simulink model "mfcm_siso_sim"  (Simulink 6.1)
settings: Solver=VariableStepDiscrete  StartTime=0.0  StopTime=150000  RelTol=1e-3
values from neighbouring files (symbols this model uses):
  j = find(xLabel==')')    [sdspfscope2_r13.m]
undefined symbols (not defined in the file or in its folder): calc_path_data
libraries: xbsIndex_r4 x23, simulink x5, xbsCopyrightNotice_r4 x1, xrbsComm_r4 x1, dspsigops x1, dspmathops x1
settings Model: Creator=singhj  LastModifiedBy=alexc
settings DebuggingCC: SolverPrmCheckMsg=warning

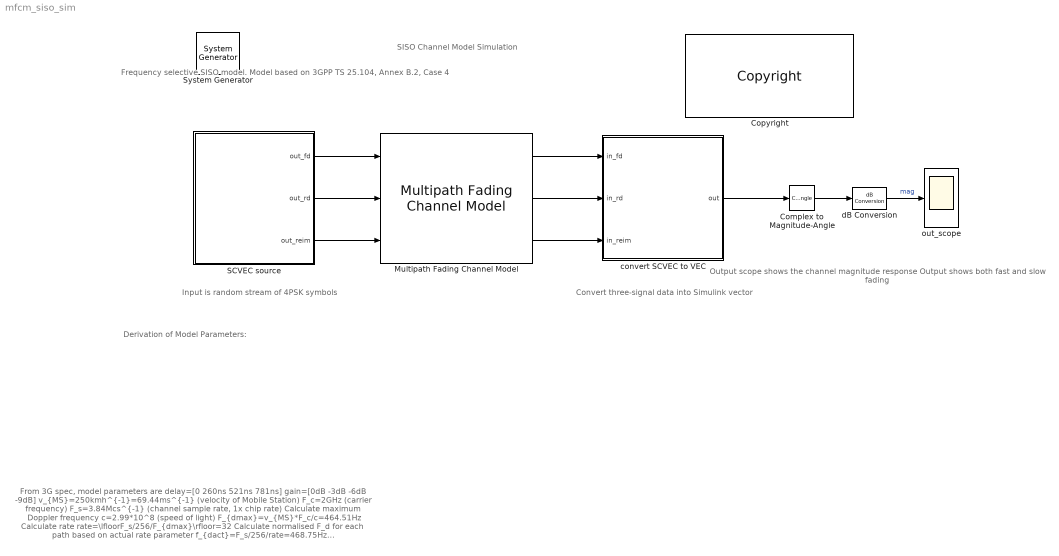
== system mfcm_siso_sim ==
  note: Output scope shows the channel magnitude response
      |
      | Output shows both fast and slow fading
  note: From 3G spec, model parameters are
      |   delay=[0 260ns 521ns 781ns]
      |   gain=[0dB -3dB -6dB -9dB]
      |   v_{MS}=250kmh^{-1}=69.44ms^{-1} (velocity of Mobile Station)
      |   F_c=2GHz (carrier frequency)
      |   F_s=3.84Mcs^{-1} (channel sample rate, 1x chip rate)
      |
      | Calculate maximum Doppler frequency
      |   c=2.99*10^8 (speed of light)
      |   F_{dmax}=v_{MS}*F_c/c=464.51Hz
      |
      | Calculate rate
      |   rate=\lfloorF_s/256/F_{dmax}\rfloor=32
      |
      | Calculate normalised F_d for each path based on actual rate parameter
      |   f_{dact}=F_s/256/rate=468.75Hz
      |   f_d=F_{dmax}/F_{dact}=0.990
      |
      | This can be passed as the second parameter of 'calc\_path\_data' to correct for the small difference between specified and actual F_d
      |   calc\_path\_data(ones(1,1,4)*2,0.990)
      |
      | Convert the delay vector to sample indexes
      |   delay_{sam}=round(delay*F_s)=[0 1 2 3]
      |
      | Convert the gain vector from dB to linear
      |   gain_{linear}=10^{gain/10}=[1.000 0.5012 0.2512 0.1259]
  note: SISO Channel Model Simulation
  note: Input is random stream of 4PSK symbols
  note: Convert three-signal data into
      | Simulink vector
  note: Frequency selective SISO model. Model based on 3GPP TS 25.104, Annex B.2, Case 4
  note: Derivation of Model Parameters:
  " System Generator" : xbsIndex_r4/ System Generator  Tag=genX  xilinxfamily=Virtex4  part=xc4vsx25  speed=-11  package=ff668  synthesis_tool=XST  directory=./netlist  testbench=off  simulink_period=1  sysclk_period=5  incr_netlist=off  trim_vbits=Everywhere in SubSystem  dbl_ovrd=According to Block Masks  core_generation=According to Block Masks  run_coregen=off  deprecated_control=off  eval_field=0  block_type=sysgen
  Complex to Magnitude-Angle : ComplexToMagnitudeAngle  Output=Magnitude
  Copyright : xbsCopyrightNotice_r4/Copyright
  Multipath Fading Channel Model : xrbsComm_r4/Multipath Fading Channel Model  DELAY=[0; 1; 2; 3]  GAIN=10.^([0; -3; -6; -9]/10)  RT=1  RR=1  SPEC_DATA=calc_path_data(ones(1,1,4)*2,0.990)  RATE=32  DATAPATH_WIDTH=18  TX_BINPT=17  FADE_BINPT=15  RX_BINPT=15  MAT_BINPT=17  SEED='461AF8228C9F8C92'  block_type=delay
      settings: infoedit=Multipath Fading Channel Model.  block_version=VER_STRING_GOES_HERE
  SCVEC source : Subsystem  mask{DATA=exp(j*2*pi*(round(4*rand(1,8191))+0.5)/4), WIDTH=18, BINPT=17, TF=2*4*1*1*ceil(64/32), REP_FILL=Zeros, TS=1}
      mask prompts: DATA "Constant Data"; WIDTH "Output Width"; BINPT "Output Binary Point"; TF "Frame Period (fd-to-fd time)"; REP_FILL "Fill with:"; TS "Sample Period"
      mask StyleString: edit,edit,edit,edit,popup(Zeros|Data),edit
  convert SCVEC to VEC : Subsystem  mask{VEC_SIZE=1, REP=1}
      mask prompts: VEC_SIZE "Input Vector Size"; REP "Output Repetition Count"
  dB Conversion : dspmathops/dB Conversion  dBtype=dB  intype=Amplitude  R=1  fuzz=off
  out_scope : Scope
      settings: YMin=-40  YMax=20  MaxDataPoints=150000
  wires:
  Complex to Magnitude-Angle/1 -> dB Conversion/1
  dB Conversion/1 -> out_scope/1  "mag"
  SCVEC source/1(out_fd) -> Multipath Fading Channel Model/1
  SCVEC source/2(out_rd) -> Multipath Fading Channel Model/2
  SCVEC source/3(out_reim) -> Multipath Fading Channel Model/3
  convert SCVEC to VEC/1(out) -> Complex to Magnitude-Angle/1
  Multipath Fading Channel Model/1 -> convert SCVEC to VEC/1(in_fd)
  Multipath Fading Channel Model/2 -> convert SCVEC to VEC/2(in_rd)
  Multipath Fading Channel Model/3 -> convert SCVEC to VEC/3(in_reim)

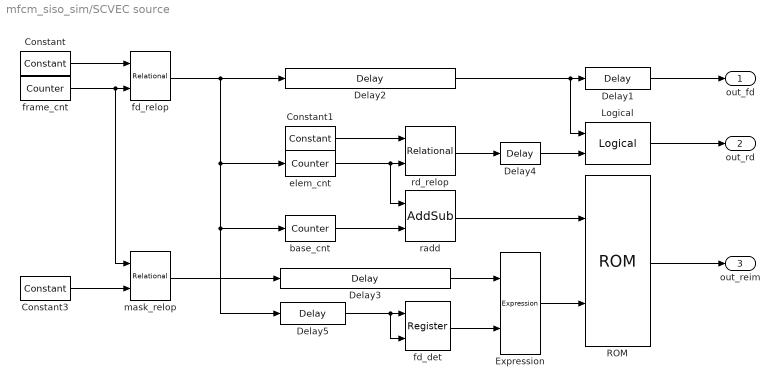
== system mfcm_siso_sim/SCVEC source ==
  Constant : xbsIndex_r4/Constant  arith_type=Unsigned  const=0  n_bits=1  bin_pt=0  explicit_period=off  period=1  equ=P=C  opselect=C  inp2=PCIN>>17  opr=+  inp1=P  carry=CIN  dbl_ovrd=off  block_type=constant
      settings: block_version=VER_STRING_GOES_HERE
  Constant1 : xbsIndex_r4/Constant  arith_type=Unsigned  const=2*size(DATA,1)-1  n_bits=ceil(log2(2*size(DATA,1)))  bin_pt=0  explicit_period=off  period=1  equ=P=C  opselect=C  inp2=PCIN>>17  opr=+  inp1=P  carry=CIN  dbl_ovrd=off  block_type=constant
      settings: block_version=VER_STRING_GOES_HERE
  Constant3 : xbsIndex_r4/Constant  arith_type=Unsigned  const=2*size(DATA,1)*double(REP_FILL==1)+TF*double(REP_FILL==2)  n_bits=1+ceil(log2(TF))  bin_pt=0  explicit_period=off  period=1  equ=P=C  opselect=C  inp2=PCIN>>17  opr=+  inp1=P  carry=CIN  dbl_ovrd=off  block_type=constant
      settings: block_version=VER_STRING_GOES_HERE
  Delay1 : xbsIndex_r4/Delay  en=off  latency=1  dbl_ovrd=off  reg_retiming=off  block_type=delay
      settings: infoedit=Hardware notes: A delay line is a chain, each link of which is an SRL16 followed by a flip-flop. If register retiming is enabled, the delay line is a chain of flip-flops.  block_version=VER_STRING_GOES_HERE
  Delay2 : xbsIndex_r4/Delay  en=off  latency=2  dbl_ovrd=off  reg_retiming=off  block_type=delay
      settings: infoedit=Hardware notes: A delay line is a chain, each link of which is an SRL16 followed by a flip-flop. If register retiming is enabled, the delay line is a chain of flip-flops.  block_version=VER_STRING_GOES_HERE
  Delay3 : xbsIndex_r4/Delay  en=off  latency=2  dbl_ovrd=off  reg_retiming=off  block_type=delay
      settings: infoedit=Hardware notes: A delay line is a chain, each link of which is an SRL16 followed by a flip-flop. If register retiming is enabled, the delay line is a chain of flip-flops.  block_version=VER_STRING_GOES_HERE
  Delay4 : xbsIndex_r4/Delay  en=off  latency=1  dbl_ovrd=off  reg_retiming=off  block_type=delay
      settings: infoedit=Hardware notes: A delay line is a chain, each link of which is an SRL16 followed by a flip-flop. If register retiming is enabled, the delay line is a chain of flip-flops.  block_version=VER_STRING_GOES_HERE
  Delay5 : xbsIndex_r4/Delay  en=off  latency=1  dbl_ovrd=off  reg_retiming=off  block_type=delay
      settings: infoedit=Hardware notes: A delay line is a chain, each link of which is an SRL16 followed by a flip-flop. If register retiming is enabled, the delay line is a chain of flip-flops.  block_version=VER_STRING_GOES_HERE
  Expression : xbsIndex_r4/Expression  expression=a & ~b  align_bp=on  en=off  latency=1  precision=Full  arith_type=Unsigned  n_bits=16  bin_pt=0  dbl_ovrd=off  block_type=expr
      settings: block_version=VER_STRING_GOES_HERE
  Logical : xbsIndex_r4/Logical  logical_function=OR  inputs=2  en=off  latency=1  precision=Full  arith_type=Unsigned  n_bits=16  bin_pt=0  align_bp=on  dbl_ovrd=off  block_type=logical
      settings: block_version=VER_STRING_GOES_HERE
  ROM : xbsIndex_r4/ROM  depth=2^ceil(log2(2*numel(DATA)))  initVector=reshape([real(reshape(DATA,1,[])); imag(reshape(DATA,1,[]))],[],1)  distributed_mem=Block RAM  rst=on  init_reg=0  en=off  latency=1  arith_type="Signed  (2's comp)"  n_bits=WIDTH  bin_pt=BINPT  dbl_ovrd=off  use_rpm=on  block_type=sprom
      settings: block_version=VER_STRING_GOES_HERE
  base_cnt : xbsIndex_r4/Counter  cnt_type=Free Running  cnt_to=Inf  operation=Up  start_count=-2*size(DATA,1)  cnt_by_val=2*size(DATA,1)  arith_type=Unsigned  n_bits=ceil(log2(2*numel(DATA)))  bin_pt=0  load_pin=off  rst=off  en=on  dbl_ovrd=off  explicit_period=off  period=1  use_behavioral_HDL=off  use_rpm=off  block_type=counter
      settings: block_version=VER_STRING_GOES_HERE
  elem_cnt : xbsIndex_r4/Counter  cnt_type=Count Limited  cnt_to=2*size(DATA,1)-1  operation=Up  start_count=0  cnt_by_val=1  arith_type=Unsigned  n_bits=ceil(log2(2*size(DATA,1)))  bin_pt=0  load_pin=off  rst=on  en=off  dbl_ovrd=off  explicit_period=off  period=1  use_behavioral_HDL=off  use_rpm=off  block_type=counter
      settings: block_version=VER_STRING_GOES_HERE
  fd_det : xbsIndex_r4/Register  init=0  rst=off  en=on  dbl_ovrd=off  block_type=register
      settings: block_version=VER_STRING_GOES_HERE
  fd_relop : xbsIndex_r4/Relational  mode=a=b  en=off  latency=1  dbl_ovrd=off  block_type=relational
      settings: block_version=VER_STRING_GOES_HERE
  frame_cnt : xbsIndex_r4/Counter  cnt_type=Count Limited  cnt_to=TF-1  operation=Up  start_count=0  cnt_by_val=1  arith_type=Unsigned  n_bits=ceil(log2(TF))  bin_pt=0  load_pin=off  rst=off  en=off  dbl_ovrd=off  explicit_period=off  period=TS  use_behavioral_HDL=off  use_rpm=off  block_type=counter
      settings: block_version=VER_STRING_GOES_HERE
  mask_relop : xbsIndex_r4/Relational  mode=a>=b  en=off  latency=1  dbl_ovrd=off  block_type=relational
      settings: block_version=VER_STRING_GOES_HERE
  radd : xbsIndex_r4/AddSub  mode=Addition  use_carryin=off  use_carryout=off  en=off  latency=1  precision=User Defined  arith_type=Unsigned  n_bits=ceil(log2(2*numel(DATA)))  bin_pt=0  quantization=Truncate  overflow=Wrap  dbl_ovrd=off  use_behavioral_HDL=off  pipelined=off  use_rpm=on  block_type=addsub
      settings: block_version=VER_STRING_GOES_HERE
  rd_relop : xbsIndex_r4/Relational  mode=a=b  en=off  latency=1  dbl_ovrd=off  block_type=relational
      settings: block_version=VER_STRING_GOES_HERE
  out_fd : Outport
  out_rd : Outport  Port=2
  out_reim : Outport  Port=3
  wires:
  fd_det/1 -> Expression/2
  Delay3/1 -> Expression/1
  Delay5/1 -> fd_det/2, fd_det/1
  Delay4/1 -> Logical/2
  Delay1/1 -> out_fd/1
  Expression/1 -> ROM/2
  mask_relop/1 -> Delay3/1
  Constant3/1 -> mask_relop/2
  Logical/1 -> out_rd/1
  base_cnt/1 -> radd/2
  radd/1 -> ROM/1
  elem_cnt/1 -> radd/1, rd_relop/2
  Delay2/1 -> Logical/1, Delay1/1
  rd_relop/1 -> Delay4/1
  Constant1/1 -> rd_relop/1
  ROM/1 -> out_reim/1
  fd_relop/1 -> Delay2/1, Delay5/1, base_cnt/1, elem_cnt/1
  frame_cnt/1 -> mask_relop/1, fd_relop/2
  Constant/1 -> fd_relop/1

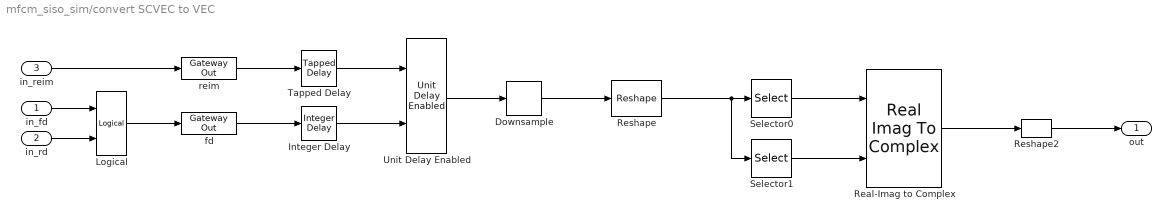
== system mfcm_siso_sim/convert SCVEC to VEC ==
  in_fd : Inport  Port=1  LatchInput=off
  in_rd : Inport  Port=2  LatchInput=off
  in_reim : Inport  Port=3  LatchInput=off
  Downsample : dspsigops/Downsample  N=2*VEC_SIZE*REP  phase=0  ic=0  smode=Allow multirate  fmode=Maintain input frame size
  Integer Delay : simulink/Discrete/Integer Delay  vinit=0.0  samptime=-1  NumDelays=2*VEC_SIZE
  Logical : xbsIndex_r4/Logical  logical_function=AND  inputs=2  en=off  latency=0  precision=Full  arith_type=Unsigned  n_bits=8  bin_pt=2  align_bp=on  dbl_ovrd=off  block_type=logical
      settings: xl_area=[0, 0, 0, 0, 0, 0, 0]  block_version=VER_STRING_GOES_HERE
  Real-Imag to Complex : RealImagToComplex
  Reshape : simulink/Math Operations/Reshape  OutputDimensionality=Customize  OutputDimensions=[2,VEC_SIZE]
  Reshape2 : simulink/Math Operations/Reshape  OutputDimensionality=1-D array  OutputDimensions=[2,VEC_SIZE]
  Selector0 : Selector  InputType=Matrix  Elements=[1 3]  Columns=-1  InputPortWidth=3
  Selector1 : Selector  InputType=Matrix  Elements=[1 3]  Rows=2  Columns=-1  InputPortWidth=3
  Tapped Delay : simulink/Discrete/Tapped Delay  vinit=0.0  samptime=-1  NumDelays=2*VEC_SIZE  DelayOrder=Oldest  includeCurrent=off
  Unit Delay Enabled : simulink/Additional Math & Discrete/Additional Discrete/Unit Delay Enabled  vinit=0.0  tsamp=-1
  fd : xbsIndex_r4/Gateway Out  hdl_port=on  timing_constraint=None  locs_specified=off  LOCs={}  block_type=gatewayout
      settings: infoedit="Gateway out block.  Converts Xilinx fixed point inputs into ouputs of type Simulink integer, double, or fixed point.<P><P>Hardware notes:  In hardware these blocks become top level output ports or are discarded, depending on how they are configured."  xl_area=[0, 0, 0, 0, 0, 0, 0]  block_version=VER_STRING_GOES_HERE
  reim : xbsIndex_r4/Gateway Out  hdl_port=on  timing_constraint=None  locs_specified=off  LOCs={}  block_type=gatewayout
      settings: infoedit="Gateway out block.  Converts Xilinx fixed point inputs into ouputs of type Simulink integer, double, or fixed point.<P><P>Hardware notes:  In hardware these blocks become top level output ports or are discarded, depending on how they are configured."  xl_area=[0, 0, 0, 0, 0, 0, 0]  block_version=VER_STRING_GOES_HERE
  out : Outport
  wires:
  in_rd/1 -> Logical/2
  in_fd/1 -> Logical/1
  Logical/1 -> fd/1
  in_reim/1 -> reim/1
  Reshape2/1 -> out/1
  Real-Imag to Complex/1 -> Reshape2/1
  Selector1/1 -> Real-Imag to Complex/2
  Selector0/1 -> Real-Imag to Complex/1
  Reshape/1 -> Selector1/1, Selector0/1
  Downsample/1 -> Reshape/1
  Unit Delay Enabled/1 -> Downsample/1
  Tapped Delay/1 -> Unit Delay Enabled/1
  Integer Delay/1 -> Unit Delay Enabled/2
  fd/1 -> Integer Delay/1
  reim/1 -> Tapped Delay/1
